simulink model "delta_coils"  (R2021a)
settings: Solver=VariableStepAuto  StartTime=0.0  StopTime=0.1  RelTol=1e-3
values from neighbouring files (symbols this model uses):
  fo = 50    [param.m]
  fsw = 80e3    (= 80000)    [param.m]
  MagA_f = 5    [param.m]
  MagA_l = 0    [param.m]
  MagB_f = 5    [param.m]
  MagB_l = 0    [param.m]
  MagC_f = 5    [param.m]
  MagC_l = 0    [param.m]
  PhaseA_f = 0    [param.m]
  PhaseA_h = 0    [param.m]
  PhaseA_l = 0    [param.m]
  PhaseB_f = 0    [param.m]
  PhaseB_h = 240    [param.m]
  PhaseB_l = 120    [param.m]
  PhaseC_f = 0    [param.m]
  PhaseC_h = 120    [param.m]
  PhaseC_l = 240    [param.m]
libraries: spsACVoltageSourceLib x9, spsCurrentMeasurementLib x3, spsSeriesRLCBranchLib x3, spspowerguiLib x1
settings Model: Creator=enes_  LastModifiedBy=enes_

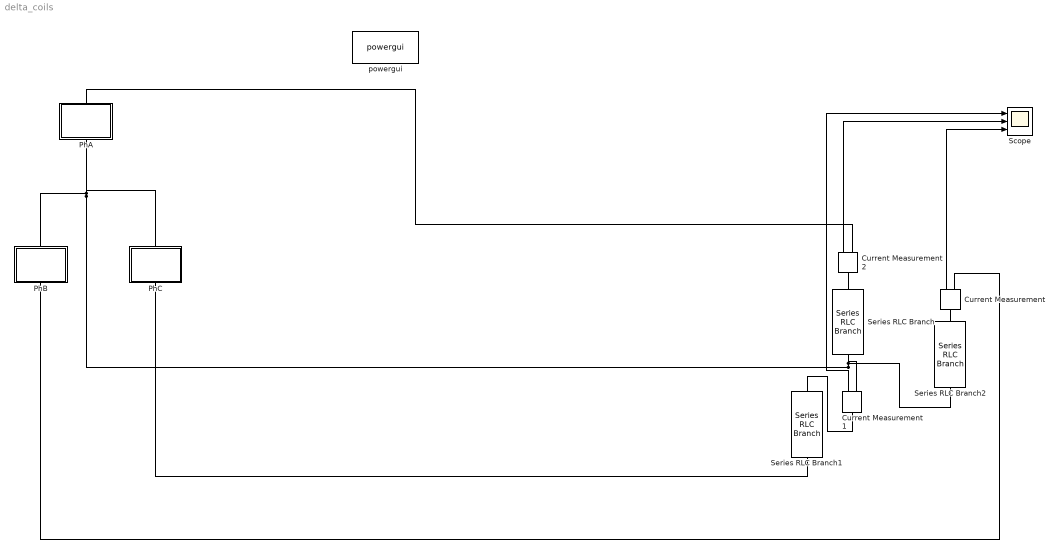
== system delta_coils ==
  Current Measurement : spsCurrentMeasurementLib/Current Measurement  PhasorSimulation=off  OutputType=Complex  PSBequivalent=0
  Current Measurement1 : spsCurrentMeasurementLib/Current Measurement  PhasorSimulation=off  OutputType=Complex  PSBequivalent=0
  Current Measurement2 : spsCurrentMeasurementLib/Current Measurement  PhasorSimulation=off  OutputType=Complex  PSBequivalent=0
  PhA : Subsystem
  PhB : Subsystem
  PhC : Subsystem
  Scope : Scope  NumInputPorts=3
  Series RLC Branch : spsSeriesRLCBranchLib/Series RLC Branch  LConnTagsString=__new0  RConnTagsString=__new0  BranchType=R  Resistance=1  Inductance=1e-3  SetiL0=off  InitialCurrent=0  Capacitance=1e-6  Setx0=off  InitialVoltage=0  Measurements=None
  Series RLC Branch1 : spsSeriesRLCBranchLib/Series RLC Branch  LConnTagsString=__new0  RConnTagsString=__new0  BranchType=R  Resistance=1  Inductance=1e-3  SetiL0=off  InitialCurrent=0  Capacitance=1e-6  Setx0=off  InitialVoltage=0  Measurements=None
  Series RLC Branch2 : spsSeriesRLCBranchLib/Series RLC Branch  LConnTagsString=__new0  RConnTagsString=__new0  BranchType=R  Resistance=1  Inductance=1e-3  SetiL0=off  InitialCurrent=0  Capacitance=1e-6  Setx0=off  InitialVoltage=0  Measurements=None
  powergui : spspowerguiLib/powergui  Priority=1  SimulationMode=Discrete  SampleTime=1e-7  frequency=60  Iterations=50  frequencyindice=79900  Pbase=100e6  ErrMax=1e-4  UnitsV=kV  UnitsW=MW  buscounter=0  FunctionMessages=off  echomessages=off  EnableUseOfTLC=off  CurrentSourceSwitches=off  DisableSnubberDevices=off  DisableRonSwitches=off  DisableVfSwitches=off  DisplayEquations=off  AutomaticDiscreteSolvers=off  SolverType=Tustin/Backward Euler (TBE)  Interpol=off  ExternalGateDelay=off  methode=off  Ts=100  x0status=blocks  SPID=on  SwTol=0  HookPort=off  NonlinearTolerance=1e-4  nMaxIteration=100  ContinueOnMaxIteration=off  RestoreLinks=warning  ResistiveCurrentMeasurement=off  Frange=[0:2:500]  Ylog=off  Xlog=on  ShowGrid=off  save=off  variable=ZData  structure=0  ZoomFFT=off  StartTime=0.0  cycles=1  DisplayStyle=1  fundamental=60  FreqAxis=off  MaxFrequency=1000  frequencyindicesteady=1  RmsSteady=1  display=off
  wires:
  Current Measurement/1 -> Scope/3
  Current Measurement2/1 -> Scope/2
  Current Measurement1/1 -> Scope/1
  connections:
  Series RLC Branch/RConn1 -- Series RLC Branch2/RConn1 -- Current Measurement1/RConn1 -- PhA/LConn1 -- PhC/LConn1 -- PhB/LConn1
  Current Measurement2/RConn1 -- PhA/RConn1
  Current Measurement1/LConn1 -- Series RLC Branch1/LConn1
  Current Measurement2/LConn1 -- Series RLC Branch/LConn1
  Current Measurement/LConn1 -- Series RLC Branch2/LConn1
  Series RLC Branch1/RConn1 -- PhC/RConn1
  Current Measurement/RConn1 -- PhB/RConn1

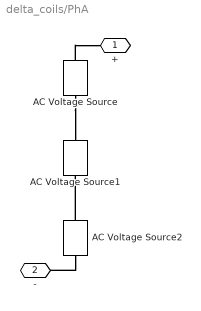
== system delta_coils/PhA ==
  AC Voltage Source : spsACVoltageSourceLib/AC Voltage Source  Amplitude=MagA_l  Phase=PhaseA_l  Frequency=fsw-2*fo  SampleTime=0  Measurements=None  BusType=swing  Pref=10e3  Qref=0  Qmin=-inf  Qmax=+inf
  AC Voltage Source1 : spsACVoltageSourceLib/AC Voltage Source  Amplitude=MagA_f  Phase=PhaseA_f  Frequency=fsw  SampleTime=0  Measurements=None  BusType=swing  Pref=10e3  Qref=0  Qmin=-inf  Qmax=+inf
  AC Voltage Source2 : spsACVoltageSourceLib/AC Voltage Source  Amplitude=MagA_l  Phase=PhaseA_h  Frequency=fsw+2*fo  SampleTime=0  Measurements=None  BusType=swing  Pref=10e3  Qref=0  Qmin=-inf  Qmax=+inf
  + : PMIOPort  Side=Right
  - : PMIOPort  Port=2  Side=Left
  connections:
  AC Voltage Source/LConn1 -- AC Voltage Source1/RConn1
  AC Voltage Source2/LConn1 -- -/RConn1
  AC Voltage Source/RConn1 -- +/RConn1
  AC Voltage Source2/RConn1 -- AC Voltage Source1/LConn1

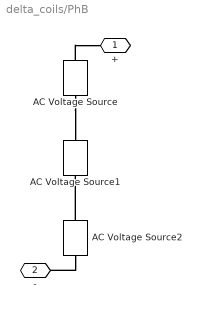
== system delta_coils/PhB ==
  AC Voltage Source : spsACVoltageSourceLib/AC Voltage Source  Amplitude=MagB_l  Phase=PhaseB_l  Frequency=fsw-2*fo  SampleTime=0  Measurements=None  BusType=swing  Pref=10e3  Qref=0  Qmin=-inf  Qmax=+inf
  AC Voltage Source1 : spsACVoltageSourceLib/AC Voltage Source  Amplitude=MagB_f  Phase=PhaseB_f  Frequency=fsw  SampleTime=0  Measurements=None  BusType=swing  Pref=10e3  Qref=0  Qmin=-inf  Qmax=+inf
  AC Voltage Source2 : spsACVoltageSourceLib/AC Voltage Source  Amplitude=MagB_l  Phase=PhaseB_h  Frequency=fsw+2*fo  SampleTime=0  Measurements=None  BusType=swing  Pref=10e3  Qref=0  Qmin=-inf  Qmax=+inf
  + : PMIOPort  Side=Right
  - : PMIOPort  Port=2  Side=Left
  connections:
  AC Voltage Source/LConn1 -- AC Voltage Source1/RConn1
  AC Voltage Source2/LConn1 -- -/RConn1
  AC Voltage Source/RConn1 -- +/RConn1
  AC Voltage Source2/RConn1 -- AC Voltage Source1/LConn1

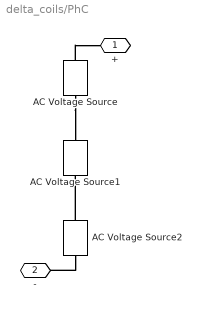
== system delta_coils/PhC ==
  AC Voltage Source : spsACVoltageSourceLib/AC Voltage Source  Amplitude=MagC_l  Phase=PhaseC_l  Frequency=fsw-2*fo  SampleTime=0  Measurements=None  BusType=swing  Pref=10e3  Qref=0  Qmin=-inf  Qmax=+inf
  AC Voltage Source1 : spsACVoltageSourceLib/AC Voltage Source  Amplitude=MagC_f  Phase=PhaseC_f  Frequency=fsw  SampleTime=0  Measurements=None  BusType=swing  Pref=10e3  Qref=0  Qmin=-inf  Qmax=+inf
  AC Voltage Source2 : spsACVoltageSourceLib/AC Voltage Source  Amplitude=MagC_l  Phase=PhaseC_h  Frequency=fsw+2*fo  SampleTime=0  Measurements=None  BusType=swing  Pref=10e3  Qref=0  Qmin=-inf  Qmax=+inf
  + : PMIOPort  Side=Right
  - : PMIOPort  Port=2  Side=Left
  connections:
  AC Voltage Source/LConn1 -- AC Voltage Source1/RConn1
  AC Voltage Source2/LConn1 -- -/RConn1
  AC Voltage Source/RConn1 -- +/RConn1
  AC Voltage Source2/RConn1 -- AC Voltage Source1/LConn1
